simulink model "Simulink_2"  (R2013b)
settings: Solver=ode45  StartTime=0.0  StopTime=50.0  RelTol=1e-3
settings Model: Creator=99900361  LastModifiedBy=99900361
settings DataIOCC: SignalLoggingSaveFormat=ModelDataLogs  SignalLoggingName=sigsOut
settings DebuggingCC: SaveWithParameterizedLinksMsg=none  SignalResolutionControl=TryResolveAllWithWarning  SolverPrmCheckMsg=none  MultiTaskDSMMsg=warning  MultiTaskCondExecSysMsg=none  StrictBusMsg=None
settings HardwareCC: TargetUnknown=on
settings RTWCC: IncludeERTFirstTime=on
settings GRTTargetCC: CombineOutputUpdateFcns=off  GRTInterface=on

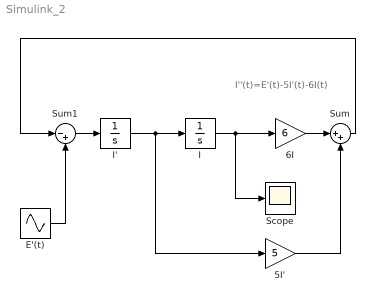
== system Simulink_2 ==
  note: I''(t)=E'(t)-5I'(t)-6I(t)
  5I' : Gain  Gain=5  SaturateOnIntegerOverflow=on  OutDataTypeStr=Inherit: Same as input  ParamDataTypeStr=Inherit: Same as input
  6I : Gain  Gain=6  SaturateOnIntegerOverflow=on  OutDataTypeStr=Inherit: Same as input  ParamDataTypeStr=Inherit: Same as input
  E'(t) : Sin  Amplitude=10  SampleTime=0
  I : Integrator  InitialCondition=1
  I' : Integrator  InitialCondition=5
  Scope : Scope
  Sum : Sum  Inputs=|++  SaturateOnIntegerOverflow=on
  Sum1 : Sum  Inputs=|-+  SaturateOnIntegerOverflow=on
  wires:
  I'/1 -> I/1, 5I'/1
  I/1 -> 6I/1, Scope/1
  6I/1 -> Sum/1
  Sum1/1 -> I'/1
  E'(t)/1 -> Sum1/2
  5I'/1 -> Sum/2
  Sum/1 -> Sum1/1
